simulink model "MotorTorqueControlTest_working_5_8_2022_ADC_FILT_Mo"  (R2024b)
settings: Solver=FixedStepAuto  StartTime=0.0  StopTime=inf  FixedStep=0.001  RelTol=1e-3  EnableMultiTasking=on
undefined symbols (not defined in the file): mu_X, mu_y, sigma_X, sigma_y
libraries: slrealtimeethercatlib x35, slrealtimeiplib x6, slrealtimeutilitieslib x5, simulink_extras x5, slrealtimeloglib x3, slpidlib x1, simulink x1
(part 3 of 4)

== matlab function MotorTorqueControlTest_working_5_8_2022_ADC_FILT_Mo/pack_data ==
  data: p_all input; x output; IMU_all input; angle input; phase input; p_min input; p_max input
function x = pack_data(p_all, IMU_all, angle, phase, p_min, p_max)
% Compute derived pressure features


p_heel = max(p_all([2,7]));
p_arc  = p_all(5);
p_meta = max(p_all([3,4,8]));
p_toe  = max(p_all([1,6]));
p_sum = sum(p_all);

%% Normalize pressure features
denom = p_max - p_min;
p_heel_norm = (p_heel - p_min) / denom;
p_arc_norm  = (p_arc  - p_min) / denom;
p_meta_norm = (p_meta - p_min) / denom;
p_toe_norm  = (p_toe  - p_min) / denom;
p_sum_norm = (p_sum - p_min) / denom;



% Compute acceleration magnitude (aM) from IMU measurements (assume first three are acceleration)
aM = sqrt(sum(IMU_all(1:3).^2));

% x = [angle, p_heel_norm, p_arc_norm, p_meta_norm, p_toe_norm, p_sum_norm, IMU_all(1), IMU_all(2), IMU_all(3), aM, phase]';

% x = [angle, p_heel_norm, p_arc_norm, p_meta_norm, p_toe_norm, p_sum_norm, IMU_all(2), phase]';
x = [p_heel_norm, p_arc_norm, p_meta_norm, p_toe_norm, p_sum_norm, IMU_all(2), phase]';

== matlab function MotorTorqueControlTest_working_5_8_2022_ADC_FILT_Mo/MATLAB Function ==
  data: SV_target_curr input; SV_target_next output; Uc_all_one input; Uc_non_one input; step_up input; step_down input; SV_target_min input; SV_target_max input; heel_strike input; assist_level input; min_cycles input; assist_threshold input
function SV_target_next = update_target_sv( ...
    SV_target_curr, ...
    Uc_all_one, Uc_non_one, ...
    step_up, step_down, ...
    SV_target_min, SV_target_max, ...
    heel_strike, ...
    assist_level, ...
    min_cycles, ...
    assist_threshold) %#codegen

    persistent cycles_assist

    if isempty(cycles_assist)
        cycles_assist = 0;
    end

    SV_target_next = SV_target_curr;

    if heel_strike == 0
        return
    end

    % Update internal assistance-cycle counter at heel strike
    if assist_level > assist_threshold
        cycles_assist = cycles_assist + 1;
    else
        cycles_assist = 0;
    end

    % Increase rule remains unchanged
    if Uc_all_one > 0.5
        SV_target_next = SV_target_curr + step_up;

    % Decrease only allowed if assistance has remained above
    % assist_threshold for at least min_cycles cycles
    elseif Uc_non_one > 0.5 && cycles_assist >= min_cycles
        SV_target_next = SV_target_curr - step_down;
    end

    % Clamp to bounds
    if SV_target_next > SV_target_max
        SV_target_next = SV_target_max;
    elseif SV_target_next < SV_target_min
        SV_target_next = SV_target_min;
    end
end

== matlab function MotorTorqueControlTest_working_5_8_2022_ADC_FILT_Mo/SV Estimator/circBuffer2 ==
  data: updated_SV output; SV input; heel_strike input
function updated_SV = circbuffer(SV, heel_strike)
%#codegen
% SV          : current sample value (scalar)
% heel_strike : logical/boolean flag
% updated_SV  : mean of 2-sample circular buffer

    persistent buf idx
    
    % Initialize persistent variables on first call
    if isempty(buf)
        % 2‑element buffer, same type as SV
        buf = zeros(1, 30, 'like', SV);
        idx = 1;
    end

    % Update buffer only on heel strike
    if heel_strike
        buf(idx) = SV;
        idx = rem(idx, 2) + 1;   % cycles 1 → 2 → 1 → 2 ...
    end

    % Output mean of buffer
    % (equivalent to mean(buf) but explicit for clarity)
    updated_SV = (buf(1) + buf(2)) / 2;
end

== matlab function MotorTorqueControlTest_working_5_8_2022_ADC_FILT_Mo/MATLAB Function3 ==
  data: Uc input; window_len_up input; window_len_down input; heel_strike input; Uc_buffer input; Uc_count input; Uc_all_one output; Uc_non_one output; Uc_buffer_next output; Uc_count_next output
function [Uc_all_one, Uc_non_one, Uc_buffer_next, Uc_count_next] = calculate_Uc_hist( ...
    Uc, window_len_up, window_len_down, heel_strike, Uc_buffer, Uc_count) %#codegen
% Uc_all_one: 1 if >=90% of last window_len_up samples are 1
% Uc_non_one: 1 if >=90% of last window_len_down samples are NOT 1
% IMPORTANT: heel_strike must be a 1-sample pulse (rising-edge event).
% Resets (buffer + BOTH counters) whenever either flag triggers (SV updated).

    % ---- Fixed output types/sizes ----
    Uc_all_one      = 0.0;
    Uc_non_one      = 0.0;

    Uc_buffer_next  = zeros(60,1,'like',Uc_buffer);
    Uc_buffer_next(:) = Uc_buffer(1:60);

    Uc_count_next   = zeros(2,1,'like',Uc_count);
    Uc_count_next(:)= Uc_count(1:2);

    % ---- Clamp window lengths to [1,60] ----
    Nup = int32(floor(window_len_up));
    if Nup < 1,  Nup = int32(1);  elseif Nup > 60, Nup = int32(60); end

    Ndn = int32(floor(window_len_down));
    if Ndn < 1,  Ndn = int32(1);  elseif Ndn > 60, Ndn = int32(60); end

    % ---- Use ONE shared count (stored in both elements for compatibility) ----
    count = int32(Uc_count_next(1));
    if count < 0
        count = int32(0);
    elseif count > 60
        count = int32(60);
    end

    % ---- Update buffer + count ONLY at heel strike pulse ----
    if heel_strike ~= 0
        Uc_buffer_next(1:end-1) = Uc_buffer_next(2:end);
        Uc_buffer_next(end)     = Uc;

        if count < 60
            count = count + 1;
        end
    end

    % Write count back (both entries same)
    Uc_count_next(1) = cast(count,'like',Uc_count_next(1));
    Uc_count_next(2) = cast(count,'like',Uc_count_next(2));

    tol = 1e-6; % if your Uc is "almost 1" (e.g., 0.999), increase this (e.g., 1e-3)

    % ---- Evaluate BOTH flags from the same buffer snapshot ----
    trig_up = false;
    trig_dn = false;

    % ===== UP: all-one =====
    if count >= Nup
        idx0 = int32(61) - Nup;       % 60 - Nup + 1
        oneCount = int32(0);
        for i = idx0:int32(60)
            if Uc_buffer_next(i) >= (1 - tol)
                oneCount = oneCount + 1;
            end
        end
        need90 = idivide(int32(9)*Nup + int32(9), int32(10), 'floor'); % ceil(0.9*Nup)
        if oneCount >= need90
            Uc_all_one = 1.0;
            trig_up = true;
        end
    end

    % ===== DOWN: non-one =====
    if count >= Ndn
        idx0 = int32(61) - Ndn;
        oneCount = int32(0);
        for i = idx0:int32(60)
            if Uc_buffer_next(i) >= (1 - tol)
                oneCount = oneCount + 1;
            end
        end
        need90 = idivide(int32(9)*Ndn + int32(9), int32(10), 'floor'); % ceil(0.9*Ndn)
        if (Ndn - oneCount) >= need90
            Uc_non_one = 1.0;
            trig_dn = true;
        end
    end

    % ---- Reset AFTER any trigger (SV updated), regardless of direction ----
    if trig_up || trig_dn
        Uc_buffer_next(:) = 0;
        count = int32(0);
        Uc_count_next(1) = cast(count,'like',Uc_count_next(1));
        Uc_count_next(2) = cast(count,'like',Uc_count_next(2));
    end
end

== matlab function MotorTorqueControlTest_working_5_8_2022_ADC_FILT_Mo/update_target_sv_mean_assistance ==
  data: SV_target_curr input; SV_target_next output; Uc_all_one input; Uc_non_one input; step_up input; step_down input; SV_target_min input; SV_target_max input; heel_strike input; assist_level input; min_cycles input; assist_threshold input
function SV_target_next = update_target_sv( ...
    SV_target_curr, ...
    Uc_all_one, Uc_non_one, ...
    step_up, step_down, ...
    SV_target_min, SV_target_max, ...
    heel_strike, ...
    assist_level, ...
    min_cycles, ...
    assist_threshold) %#codegen

    persistent assist_hist hist_count

    if isempty(assist_hist)
        assist_hist = zeros(30,1);   % store up to last 30 cycles
        hist_count   = 0;
    end

    SV_target_next = SV_target_curr;

    if heel_strike == 0
        return
    end

    % Make sure min_cycles stays within valid range [1, 30]
    window_len = round(min_cycles);
    if window_len < 1
        window_len = 1;
    elseif window_len > 30
        window_len = 30;
    end

    % Update assistance history at heel strike
    if hist_count < 30
        hist_count = hist_count + 1;
        assist_hist(hist_count) = assist_level;
    else
        assist_hist(1:29) = assist_hist(2:30);
        assist_hist(30)   = assist_level;
    end

    % Increase rule remains unchanged
    if Uc_all_one > 0.5
        SV_target_next = SV_target_curr + step_up;

    % Decrease rule uses mean of last min_cycles assistance values
    elseif Uc_non_one > 0.5 && hist_count >= window_len
        sum_assist = 0;
        for k = hist_count-window_len+1 : hist_count
            sum_assist = sum_assist + assist_hist(k);
        end
        mean_assist = sum_assist / window_len;

        if mean_assist > assist_threshold
            SV_target_next = SV_target_curr - step_down;
        end
    end

    % Clamp to bounds
    if SV_target_next > SV_target_max
        SV_target_next = SV_target_max;
    elseif SV_target_next < SV_target_min
        SV_target_next = SV_target_min;
    end
end

== matlab function MotorTorqueControlTest_working_5_8_2022_ADC_FILT_Mo/MATLAB Function1 ==
  data: heel_strike input; error input; gamma input; a output; gain input; a input
function a = ILC(heel_strike, error, gamma, gain, a)
    if heel_strike
        error = max(0, error);
        a = gamma * a + gain * error;
    
        if a > 10
            a = 10;
        elseif a < 0
            a = 0;
        end
    end
end

== matlab function MotorTorqueControlTest_working_5_8_2022_ADC_FILT_Mo/SV Estimator/SV_Estimator1 ==
  data: curTime input; strideSV output; data input; data_filtered input; SL output; thr_sum_FC input; thr_sum_LC input; min_event_dt input; pSum output; reset input; is_active output
function [strideSV, SL, pSum, is_active] = ...
    SV_Estimator(curTime, data, data_filtered, ...
                 thr_sum_FC, thr_sum_LC, ...
                 min_event_dt, reset) %#codegen
% Online stride-velocity estimator (pressure envelope + minAcc ZUPT)
%
% INPUT
%   data         : row-vector (width ≥ 14). May be single or double.
%                  data(1)     = time stamp (s)
%                  data(12:14) = IMU accel channels (device frame)
%   data_filtered: row-vector with pressure channels in 1:8 (here)
%   thr_sum_FC   : threshold on pSum for foot contact (FC)
%   thr_sum_LC   : threshold on pSum for foot off / load removal (LC)
%   min_event_dt : minimum time between FC / LC events (s)
%   reset        : scalar logical/0-1. When non-zero, ALL internal state is reset.
%
% OUTPUT
%   strideSV     : stride-mean velocity (m/s)
%   SL           : stride length (m)
%   pSum         : current pressure envelope (for plotting/tuning)
%   is_active    : logical flag, 1 when current estimate is considered usable.
%                  After any reset or error, this stays 0 for 3 calls.

% ------------------------------------------------------------------
% default outputs
strideSV  = 0.0;
SL        = 0.0;
pSum      = 0.0;
is_active = false;

% ------------------------------------------------------------------
% fixed parameters (internal)
g_NJ         = 9.80665;      % gravity (m/s²)
BUFFER       = 5000;         % ring-buffer length
MAX_STRIDE_T = 3.0;          % max LC→LC stride time (s)
ALPHA_FF     = 0.6;          % fraction of stance peak for FF gate
SEP_MIN      = 0.50;         % min time separation for FC/LC FSM transitions
MAX_SV       = 2.0;          % reset if strideSV > 2 m/s (safety)

% external reset flag for this call
doReset = (reset ~= 0);

% ------------------------------------------------------------------
% persistent state
persistent buf               % 11 × BUFFER: accel, vel, pos, time
persistent pEnvBuf           % 1 × BUFFER : pressure envelope (pSum)
persistent iter
persistent FC_iter LC_iter
persistent FC_idx  LC_idx
persistent SL_p strideSV_p
persistent pSum_prev tFC tLC
persistent cooldownSteps     % ≥0: remaining steps where is_active = false

% buf rows
ROW_AX=1; ROW_AY=2; ROW_AZ=3; ROW_AM=4;
ROW_VX=5; ROW_VY=6; ROW_VZ=7;
ROW_PX=8; ROW_PY=9; ROW_PZ=10; ROW_T=11;

% ------------------------------------------------------------------
% FIRST-CALL OR EXTERNAL RESET INITIALIZATION
if isempty(iter) || doReset
    buf      = zeros(11,BUFFER);
    pEnvBuf  = zeros(1,BUFFER);
    iter     = 1;

    FC_iter  = 0;
    LC_iter  = 0;
    FC_idx   = ones(1,2);
    LC_idx   = ones(1,2);

    SL_p       = 0;
    strideSV_p = 0;

    pSum_prev  = 0;
    tFC        = [-inf -inf];
    tLC        = [-inf -inf];

    % start (or restart) 3-step inactive window after reset
    cooldownSteps = 3;
end

% ------------------------------------------------------------------
% decode current packet (pressure + accel)
pressure = double(data_filtered);
IMU_data = double(data);

% keep the same heel/toe grouping for pSum as your original code
pHeel = max( pressure([2 7 8]) );
pToe  = max( pressure([1 3 4 5 6]) );
pSum  = pHeel + 1.5 * pToe;      % envelope

ax = -IMU_data(3);
ay =  IMU_data(1);
az = -IMU_data(2);

% ------------------------------------------------------------------
% gait-event detector (FC/LC from pSum)
isFC = (pSum_prev <= thr_sum_FC) && (pSum >  thr_sum_FC) ...
       && (curTime - tFC(2) > min_event_dt);
isLC = (pSum_prev >  thr_sum_LC) && (pSum <= thr_sum_LC) ...
       && (curTime - tLC(2) > min_event_dt);

if isFC
    tFC = [tFC(2) curTime];
end
if isLC
    tLC = [tLC(2) curTime];
end

pSum_prev = pSum;

% ------------------------------------------------------------------
% store current sample in buffers
idx = iter;

axg = ax * g_NJ;
ayg = ay * g_NJ;
azg = az * g_NJ;

buf(ROW_AX,idx) = axg;
buf(ROW_AY,idx) = ayg;
buf(ROW_AZ,idx) = azg;
buf(ROW_AM,idx) = sqrt(axg*axg + ayg*ayg + azg*azg);
buf(ROW_T ,idx) = curTime;

pEnvBuf(idx) = pSum;

% ------------------------------------------------------------------
% update simple FC / LC finite-state machines
if isFC
    if FC_iter==0
        FC_idx(1) = idx;
        FC_iter   = 1;
    elseif FC_iter==1 && (curTime - buf(ROW_T,FC_idx(1)) > SEP_MIN)
        FC_idx(2) = idx;
        FC_iter   = 2;
    elseif FC_iter==2 && (curTime - buf(ROW_T,FC_idx(2)) > SEP_MIN)
        FC_idx(1) = idx;
        FC_iter   = 1;
        LC_iter   = 0;
    end
end

if isLC && FC_iter>=1
    if LC_iter==0
        LC_idx(1) = idx;
        LC_iter   = 1;
    elseif LC_iter==1 && (curTime - buf(ROW_T,LC_idx(1)) > SEP_MIN)
        LC_idx(2) = idx;
        LC_iter   = 2;
    elseif LC_iter==2 && (curTime - buf(ROW_T,LC_idx(2)) > SEP_MIN)
        FC_iter   = 0;
        LC_iter   = 0;
    end
end

% ------------------------------------------------------------------
% stride finished?  (two FCs and two LCs available)
if FC_iter==2 && LC_iter==2
    fc0 = FC_idx(1); fc1 = FC_idx(2);
    lc0 = LC_idx(1); lc1 = LC_idx(2);

    % LC-to-LC stride duration
    dtLC = buf(ROW_T,lc1) - buf(ROW_T,lc0);

    % sanity check on stride duration
    if dtLC <= 0 || dtLC > MAX_STRIDE_T
        % invalid stride: don't update SL_p / strideSV_p, reset FSM
        FC_iter = 0;
        LC_iter = 0;

        % mark error → 3-step inactive window
        cooldownSteps = 3;

    else
        % ----------------------------------------------------------
        % 1) compute stance peaks for each stance (fc0→lc0, fc1→lc1)
        pPeak0 = 0;
        k      = fc0;
        while true
            v = pEnvBuf(k);
            if v > pPeak0
                pPeak0 = v;
            end
            if k == lc0, break; end
            k = adv(k, BUFFER);
        end

        pPeak1 = 0;
        k      = fc1;
        while true
            v = pEnvBuf(k);
            if v > pPeak1
                pPeak1 = v;
            end
            if k == lc1, break; end
            k = adv(k, BUFFER);
        end

        thrFF0 = ALPHA_FF * pPeak0;
        thrFF1 = ALPHA_FF * pPeak1;

        % 2) pick ZUPT indices using minAcc inside high-pressure window
        [sIdx, ~] = minAccIdxHighP(fc0, lc0, thrFF0, buf, pEnvBuf, ROW_AM, BUFFER);
        [eIdx, ~] = minAccIdxHighP(fc1, lc1, thrFF1, buf, pEnvBuf, ROW_AM, BUFFER);

        % ----------------------------------------------------------
        % ORIGINAL-STYLE 2-PASS INTEGRATION WITH DRIFT REMOVAL

        % zero velocity & position at integration start
        buf(ROW_VX,sIdx) = 0;
        buf(ROW_VY,sIdx) = 0;
        buf(ROW_VZ,sIdx) = 0;
        buf(ROW_PX,sIdx) = 0;
        buf(ROW_PY,sIdx) = 0;
        buf(ROW_PZ,sIdx) = 0;

        % first pass: accel → vel
        p = sIdx;
        c = adv(p, BUFFER);
        while true
            dt_loc = buf(ROW_T,c) - buf(ROW_T,p);
            buf(ROW_VX,c) = buf(ROW_VX,p) + 0.5*(buf(ROW_AX,p)+buf(ROW_AX,c))*dt_loc;
            buf(ROW_VY,c) = buf(ROW_VY,p) + 0.5*(buf(ROW_AY,p)+buf(ROW_AY,c))*dt_loc;
            buf(ROW_VZ,c) = buf(ROW_VZ,p) + 0.5*(buf(ROW_AZ,p)+buf(ROW_AZ,c))*dt_loc;
            if c == eIdx, break; end
            p = c;
            c = adv(c, BUFFER);
        end

        dtStride = buf(ROW_T,eIdx) - buf(ROW_T,sIdx);
        if dtStride == 0
            dtStride = eps;
        end

        vxD = buf(ROW_VX,eIdx) / dtStride;
        vyD = buf(ROW_VY,eIdx) / dtStride;
        vzD = buf(ROW_VZ,eIdx) / dtStride;

        % second pass: subtract linear drift, vel → pos
        p = sIdx;
        c = adv(p, BUFFER);
        while true
            dt_loc = buf(ROW_T,c) - buf(ROW_T,p);
            tOff   = buf(ROW_T,c) - buf(ROW_T,sIdx);

            buf(ROW_VX,c) = buf(ROW_VX,c) - vxD*tOff;
            buf(ROW_VY,c) = buf(ROW_VY,c) - vyD*tOff;
            buf(ROW_VZ,c) = buf(ROW_VZ,c) - vzD*tOff;

            buf(ROW_PX,c) = buf(ROW_PX,p) + 0.5*(buf(ROW_VX,p)+buf(ROW_VX,c))*dt_loc;
            buf(ROW_PY,c) = buf(ROW_PY,p) + 0.5*(buf(ROW_VY,p)+buf(ROW_VY,c))*dt_loc;
            buf(ROW_PZ,c) = buf(ROW_PZ,p) + 0.5*(buf(ROW_VZ,p)+buf(ROW_VZ,c))*dt_loc;

            if c == eIdx, break; end
            p = c;
            c = adv(c, BUFFER);
        end

        % stride length & mean velocity
        SL_p       = sqrt(buf(ROW_PX,eIdx)^2 + buf(ROW_PY,eIdx)^2 + buf(ROW_PZ,eIdx)^2);
        strideSV_p = SL_p / dtLC;
        if strideSV_p < 0
            strideSV_p = 0;
        end

        % optional hard reset on absurdly large SV
        if strideSV_p > MAX_SV
            buf(:,:)   = 0;
            pEnvBuf(:) = 0;
            iter       = 1;

            FC_iter  = 0;
            LC_iter  = 0;
            FC_idx   = ones(1,2);
            LC_idx   = ones(1,2);

            SL_p       = 0;
            strideSV_p = 0;

            pSum_prev  = 0;
            tFC        = [-inf -inf];
            tLC        = [-inf -inf];

            % hard error reset → 3-step inactive window
            cooldownSteps = 3;
        else
            % shift FC/LC indices for next stride
            FC_idx(1) = FC_idx(2);
            FC_iter   = 1;
            LC_idx(1) = LC_idx(2);
            LC_iter   = 1;
        end
    end
end

% advance iterator in ring buffer
iter = iter + 1;
if iter > BUFFER
    iter = 1;
end

% ------------------------------------------------------------------
% update activity flag: 3-sample cooldown after reset/error
if isempty(cooldownSteps)
    cooldownSteps = 0;
end

if cooldownSteps > 0
    is_active     = false;
    cooldownSteps = cooldownSteps - 1;
else
    is_active = true;
end

% ------------------------------------------------------------------
% outputs from persistent state
strideSV = strideSV_p;
SL       = SL_p;

end  % main function

% ==================================================================
% Helper: advance index in ring buffer
function n = adv(i, BUFFER)
n = i + 1;
if n > BUFFER
    n = 1;
end
end

% ==================================================================
% Helper: min acceleration magnitude in high-pressure window
function [idxOut, usedHigh] = minAccIdxHighP(iStart, iEnd, thrP, buf, pEnvBuf, ROW_AM, BUFFER)
% Find contiguous high-pressure window and pick min|a| inside it.
% If none exists, fall back to pure minAcc over [iStart, iEnd].

% 1) Find first and last indices with pEnv > thrP
found     = false;
firstHigh = iStart;
lastHigh  = iStart;

idx = iStart;
while true
    pEnv = pEnvBuf(idx);
    if pEnv > thrP
        if ~found
            firstHigh = idx;
            found     = true;
        end
        lastHigh = idx;
    end
    if idx == iEnd, break; end
    idx = adv(idx, BUFFER);
end

if found
    % 2) min |a| inside [firstHigh, lastHigh]
    idxOut   = firstHigh;
    mAcc     = buf(ROW_AM,idxOut);
    usedHigh = true;

    idx = firstHigh;
    while true
        accMag = buf(ROW_AM,idx);
        if accMag < mAcc
            mAcc   = accMag;
            idxOut = idx;
        end
        if idx == lastHigh, break; end
        idx = adv(idx, BUFFER);
    end
else
    % 3) fallback: no high-pressure region → minAcc over whole FC-LC
    idxOut   = minAccIdx(iStart,iEnd,buf,ROW_AM,BUFFER);
    usedHigh = false;
end
end

% ==================================================================
% Helper: pure minimum acceleration magnitude between iStart and iEnd
function idxOut = minAccIdx(iStart, iEnd, buf, ROW_AM, BUFFER)
idx    = iStart;
idxOut = iStart;
mAcc   = buf(ROW_AM,idx);

while true
    accMag = buf(ROW_AM,idx);
    if accMag < mAcc
        mAcc   = accMag;
        idxOut = idx;
    end
    if idx == iEnd, break; end
    idx = adv(idx, BUFFER);
end
end

== matlab function MotorTorqueControlTest_working_5_8_2022_ADC_FILT_Mo/Stall Check ==
  data: torque_actual input; Start_Stop input; status output; isAlive output
function [status, isAlive] = TorqueWatchdog(torque_actual, Start_Stop)
% status  : 1 = stream alive, 0 = stopped or stalled
% isStall : 1 = stall detected (latched), 0 = no stall yet
%
% Uses numeric 0/1 only (no logical true/false keywords).
% Outputs are type DOUBLE to match Simulink’s default.
%
%#codegen

% ----- USER‑TUNABLE CONSTANTS -----
Ts        = 0.001;   % sample time [s]  (set to your model step)
stallTime = 0.05;    % flat‑line duration to declare stall [s]
epsTorque = 0.000006;    % minimum change that counts as “different”
% ----------------------------------

% Persistent state
persistent lastTorque timeFrozen stallDetected sensorReady
if isempty(lastTorque)
    lastTorque     = torque_actual; % initial value
    timeFrozen     = 0;
    stallDetected  = 0;   % 0 = not stalled, 1 = stalled
    sensorReady    = 0;   % 0 = waiting for first non‑zero change
end

% ----- master gate -----
if Start_Stop == 0          % external stop / reset
    status        = 0;
    isAlive       = 1;
    timeFrozen    = 0;
    stallDetected = 0;
    sensorReady   = 0;
    lastTorque    = torque_actual;
    return
end

% ----- Start_Stop == 1 -----
if sensorReady == 0         % ignore initial flat‑line until sensor moves
    if abs(torque_actual - lastTorque) > epsTorque
        sensorReady = 1;    % sensor awake
        timeFrozen  = 0;
    end
    status  = 1;            % considered alive during warm‑up
else                         % normal watchdog
    if stallDetected == 1
        status = 0;         % latched stall
    else
        if abs(torque_actual - lastTorque) < epsTorque
            timeFrozen = timeFrozen + Ts;
            if timeFrozen >= stallTime
                stallDetected = 1;
            end
        else
            timeFrozen = 0;  % any change resets timer
        end
        status = 1 - stallDetected;  % 1 if not stalled, 0 if stalled
    end
end

% second output
isAlive = 1 - stallDetected;

% update history
lastTorque = torque_actual;
end

== matlab function MotorTorqueControlTest_working_5_8_2022_ADC_FILT_Mo/MATLAB Function4 ==
  data: x input; y output; mu_X input; sigma_X input; mu_y input; add_mu_y input; sigma_y input
function y = callGP(x, mu_X, sigma_X, mu_y, add_mu_y, sigma_y)
%#codegen
y = myModelPredict(x, mu_X, sigma_X, mu_y + add_mu_y, sigma_y);

== matlab function MotorTorqueControlTest_working_5_8_2022_ADC_FILT_Mo/SV Estimator/SV_Estimator ==
  data: curTime input; strideSV output; data input; data_filtered input; SL output; thr_sum_FC input; thr_sum_LC input; min_event_dt input; pSum output; reset input; is_active output
function [strideSV, SL, pSum, is_active] = ...
    SV_Estimator(curTime, data, data_filtered, ...
                 thr_sum_FC, thr_sum_LC, ...
                 min_event_dt, reset) %#codegen
% Online stride-velocity estimator (pressure envelope + minAcc ZUPT)
%
% INPUT
%   data         : row-vector (width ≥ 14). May be single or double.
%                  data(1)     = time stamp (s)
%                  data(12:14) = IMU accel channels (device frame)
%   data_filtered: row-vector with pressure channels in 1:8 (here)
%   thr_sum_FC   : threshold on pSum for foot contact (FC)
%   thr_sum_LC   : threshold on pSum for foot off / load removal (LC)
%   min_event_dt : minimum time between FC / LC events (s)
%   reset        : scalar logical/0-1. When non-zero, ALL internal state is reset.
%
% OUTPUT
%   strideSV     : stride-mean velocity (m/s). Updated only on a plausible
%                  stride; otherwise HOLDS the previous good value.
%   SL           : stride length (m)
%   pSum         : current pressure envelope (for plotting/tuning)
%   is_active    : logical flag, 1 when current estimate is considered usable.
%                  After any reset or error, this stays 0 for 3 calls.

% ------------------------------------------------------------------
% default outputs
strideSV  = 0.0;
SL        = 0.0;
pSum      = 0.0;
is_active = false;

% ------------------------------------------------------------------
% fixed parameters (internal)
g_NJ         = 9.80665;      % gravity (m/s²)
BUFFER       = 5000;         % ring-buffer length
MAX_STRIDE_T = 3.0;          % max LC→LC stride time (s)
ALPHA_FF     = 0.6;          % fraction of stance peak for FF gate
SEP_MIN      = 0.50;         % min time separation for FC/LC FSM transitions

% >>> CHANGED (1): plausibility band replaces the MAX_SV hard-reset.
% A stride whose estimated velocity is outside this band is treated as a bad
% estimate: the estimator HOLDS its previous good output instead of publishing
% the bad value (and instead of the old reset that zeroed the output and caused
% the drop-outs to 0). The downstream smoothing block is unchanged, so the
% controller keeps the same responsiveness -- it just never sees a bad stride.
% Set SV_MAX_VALID a little above the fastest speed the wearer actually walks.
SV_MIN_VALID = 0.3;          % m/s : below this -> integration collapsed, reject
SV_MAX_VALID = 1.8;          % m/s : above this -> integration blew up,  reject

% external reset flag for this call
doReset = (reset ~= 0);

% ------------------------------------------------------------------
% persistent state
persistent buf               % 11 × BUFFER: accel, vel, pos, time
persistent pEnvBuf           % 1 × BUFFER : pressure envelope (pSum)
persistent iter
persistent FC_iter LC_iter
persistent FC_idx  LC_idx
persistent SL_p strideSV_p
persistent pSum_prev tFC tLC
persistent cooldownSteps     % ≥0: remaining steps where is_active = false

% buf rows
ROW_AX=1; ROW_AY=2; ROW_AZ=3; ROW_AM=4;
ROW_VX=5; ROW_VY=6; ROW_VZ=7;
ROW_PX=8; ROW_PY=9; ROW_PZ=10; ROW_T=11;

% ------------------------------------------------------------------
% FIRST-CALL OR EXTERNAL RESET INITIALIZATION
if isempty(iter) || doReset
    buf      = zeros(11,BUFFER);
    pEnvBuf  = zeros(1,BUFFER);
    iter     = 1;

    FC_iter  = 0;
    LC_iter  = 0;
    FC_idx   = ones(1,2);
    LC_idx   = ones(1,2);

    SL_p       = 0;
    strideSV_p = 0;

    pSum_prev  = 0;
    tFC        = [-inf -inf];
    tLC        = [-inf -inf];

    % start (or restart) 3-step inactive window after reset
    cooldownSteps = 3;
end

% ------------------------------------------------------------------
% decode current packet (pressure + accel)
pressure = double(data_filtered);
IMU_data = double(data);

% keep the same heel/toe grouping for pSum as your original code
pHeel = max( pressure([2 7 8]) );
pToe  = max( pressure([1 3 4 5 6]) );
pSum  = pHeel + 1.5 * pToe;      % envelope

ax = -IMU_data(3);
ay =  IMU_data(1);
az = -IMU_data(2);

% ------------------------------------------------------------------
% gait-event detector (FC/LC from pSum)
isFC = (pSum_prev <= thr_sum_FC) && (pSum >  thr_sum_FC) ...
       && (curTime - tFC(2) > min_event_dt);
isLC = (pSum_prev >  thr_sum_LC) && (pSum <= thr_sum_LC) ...
       && (curTime - tLC(2) > min_event_dt);

if isFC
    tFC = [tFC(2) curTime];
end
if isLC
    tLC = [tLC(2) curTime];
end

pSum_prev = pSum;

% ------------------------------------------------------------------
% store current sample in buffers
idx = iter;

axg = ax * g_NJ;
ayg = ay * g_NJ;
azg = az * g_NJ;

buf(ROW_AX,idx) = axg;
buf(ROW_AY,idx) = ayg;
buf(ROW_AZ,idx) = azg;
buf(ROW_AM,idx) = sqrt(axg*axg + ayg*ayg + azg*azg);
buf(ROW_T ,idx) = curTime;

pEnvBuf(idx) = pSum;

% ------------------------------------------------------------------
% update simple FC / LC finite-state machines
if isFC
    if FC_iter==0
        FC_idx(1) = idx;
        FC_iter   = 1;
    elseif FC_iter==1 && (curTime - buf(ROW_T,FC_idx(1)) > SEP_MIN)
        FC_idx(2) = idx;
        FC_iter   = 2;
    elseif FC_iter==2 && (curTime - buf(ROW_T,FC_idx(2)) > SEP_MIN)
        FC_idx(1) = idx;
        FC_iter   = 1;
        LC_iter   = 0;
    end
end

if isLC && FC_iter>=1
    if LC_iter==0
        LC_idx(1) = idx;
        LC_iter   = 1;
    elseif LC_iter==1 && (curTime - buf(ROW_T,LC_idx(1)) > SEP_MIN)
        LC_idx(2) = idx;
        LC_iter   = 2;
    elseif LC_iter==2 && (curTime - buf(ROW_T,LC_idx(2)) > SEP_MIN)
        FC_iter   = 0;
        LC_iter   = 0;
    end
end

% ------------------------------------------------------------------
% stride finished?  (two FCs and two LCs available)
if FC_iter==2 && LC_iter==2
    fc0 = FC_idx(1); fc1 = FC_idx(2);
    lc0 = LC_idx(1); lc1 = LC_idx(2);

    % LC-to-LC stride duration
    dtLC = buf(ROW_T,lc1) - buf(ROW_T,lc0);

    % sanity check on stride duration
    if dtLC <= 0 || dtLC > MAX_STRIDE_T
        % invalid stride: don't update SL_p / strideSV_p, reset FSM
        FC_iter = 0;
        LC_iter = 0;

        % mark error → 3-step inactive window
        cooldownSteps = 3;

    else
        % ----------------------------------------------------------
        % 1) compute stance peaks for each stance (fc0→lc0, fc1→lc1)
        pPeak0 = 0;
        k      = fc0;
        while true
            v = pEnvBuf(k);
            if v > pPeak0
                pPeak0 = v;
            end
            if k == lc0, break; end
            k = adv(k, BUFFER);
        end

        pPeak1 = 0;
        k      = fc1;
        while true
            v = pEnvBuf(k);
            if v > pPeak1
                pPeak1 = v;
            end
            if k == lc1, break; end
            k = adv(k, BUFFER);
        end

        thrFF0 = ALPHA_FF * pPeak0;
        thrFF1 = ALPHA_FF * pPeak1;

        % 2) pick ZUPT indices using minAcc inside high-pressure window
        [sIdx, ~] = minAccIdxHighP(fc0, lc0, thrFF0, buf, pEnvBuf, ROW_AM, BUFFER);
        [eIdx, ~] = minAccIdxHighP(fc1, lc1, thrFF1, buf, pEnvBuf, ROW_AM, BUFFER);

        % ----------------------------------------------------------
        % ORIGINAL-STYLE 2-PASS INTEGRATION WITH DRIFT REMOVAL

        % zero velocity & position at integration start
        buf(ROW_VX,sIdx) = 0;
        buf(ROW_VY,sIdx) = 0;
        buf(ROW_VZ,sIdx) = 0;
        buf(ROW_PX,sIdx) = 0;
        buf(ROW_PY,sIdx) = 0;
        buf(ROW_PZ,sIdx) = 0;

        % first pass: accel → vel
        p = sIdx;
        c = adv(p, BUFFER);
        while true
            dt_loc = buf(ROW_T,c) - buf(ROW_T,p);
            buf(ROW_VX,c) = buf(ROW_VX,p) + 0.5*(buf(ROW_AX,p)+buf(ROW_AX,c))*dt_loc;
            buf(ROW_VY,c) = buf(ROW_VY,p) + 0.5*(buf(ROW_AY,p)+buf(ROW_AY,c))*dt_loc;
            buf(ROW_VZ,c) = buf(ROW_VZ,p) + 0.5*(buf(ROW_AZ,p)+buf(ROW_AZ,c))*dt_loc;
            if c == eIdx, break; end
            p = c;
            c = adv(c, BUFFER);
        end

        dtStride = buf(ROW_T,eIdx) - buf(ROW_T,sIdx);
        if dtStride == 0
            dtStride = eps;
        end

        vxD = buf(ROW_VX,eIdx) / dtStride;
        vyD = buf(ROW_VY,eIdx) / dtStride;
        vzD = buf(ROW_VZ,eIdx) / dtStride;

        % second pass: subtract linear drift, vel → pos
        p = sIdx;
        c = adv(p, BUFFER);
        while true
            dt_loc = buf(ROW_T,c) - buf(ROW_T,p);
            tOff   = buf(ROW_T,c) - buf(ROW_T,sIdx);

            buf(ROW_VX,c) = buf(ROW_VX,c) - vxD*tOff;
            buf(ROW_VY,c) = buf(ROW_VY,c) - vyD*tOff;
            buf(ROW_VZ,c) = buf(ROW_VZ,c) - vzD*tOff;

            buf(ROW_PX,c) = buf(ROW_PX,p) + 0.5*(buf(ROW_VX,p)+buf(ROW_VX,c))*dt_loc;
            buf(ROW_PY,c) = buf(ROW_PY,p) + 0.5*(buf(ROW_VY,p)+buf(ROW_VY,c))*dt_loc;
            buf(ROW_PZ,c) = buf(ROW_PZ,p) + 0.5*(buf(ROW_VZ,p)+buf(ROW_VZ,c))*dt_loc;

            if c == eIdx, break; end
            p = c;
            c = adv(c, BUFFER);
        end

        % >>> CHANGED (2): compute this stride as a CANDIDATE (local vars)
        SL_new = sqrt(buf(ROW_PX,eIdx)^2 + buf(ROW_PY,eIdx)^2 + buf(ROW_PZ,eIdx)^2);
        SV_new = SL_new / dtLC;
        if SV_new < 0
            SV_new = 0;
        end

        % >>> CHANGED (3): plausibility gate + hold-last-good
        if SV_new >= SV_MIN_VALID && SV_new <= SV_MAX_VALID
            % accept: publish this stride and roll indices to the next stride
            SL_p       = SL_new;
            strideSV_p = SV_new;

            FC_idx(1) = FC_idx(2);
            FC_iter   = 1;
            LC_idx(1) = LC_idx(2);
            LC_iter   = 1;
        else
            % reject implausible stride (collapse ~0 or blow-up):
            % HOLD the last good strideSV_p / SL_p (do NOT zero) and resync the
            % FSM, exactly like the invalid-duration path above.
            FC_iter = 0;
            LC_iter = 0;

            cooldownSteps = 3;
        end
    end
end

% advance iterator in ring buffer
iter = iter + 1;
if iter > BUFFER
    iter = 1;
end

% ------------------------------------------------------------------
% update activity flag: 3-sample cooldown after reset/error
if isempty(cooldownSteps)
    cooldownSteps = 0;
end

if cooldownSteps > 0
    is_active     = false;
    cooldownSteps = cooldownSteps - 1;
else
    is_active = true;
end

% ------------------------------------------------------------------
% outputs from persistent state
strideSV = strideSV_p;
SL       = SL_p;

end  % main function

% ==================================================================
% Helper: advance index in ring buffer
function n = adv(i, BUFFER)
n = i + 1;
if n > BUFFER
    n = 1;
end
end

% ==================================================================
% Helper: min acceleration magnitude in high-pressure window
function [idxOut, usedHigh] = minAccIdxHighP(iStart, iEnd, thrP, buf, pEnvBuf, ROW_AM, BUFFER)
% Find contiguous high-pressure window and pick min|a| inside it.
% If none exists, fall back to pure minAcc over [iStart, iEnd].

% 1) Find first and last indices with pEnv > thrP
found     = false;
firstHigh = iStart;
lastHigh  = iStart;

idx = iStart;
while true
    pEnv = pEnvBuf(idx);
    if pEnv > thrP
        if ~found
            firstHigh = idx;
            found     = true;
        end
        lastHigh = idx;
    end
    if idx == iEnd, break; end
    idx = adv(idx, BUFFER);
end

if found
    % 2) min |a| inside [firstHigh, lastHigh]
    idxOut   = firstHigh;
    mAcc     = buf(ROW_AM,idxOut);
    usedHigh = true;

    idx = firstHigh;
    while true
        accMag = buf(ROW_AM,idx);
        if accMag < mAcc
            mAcc   = accMag;
            idxOut = idx;
        end
        if idx == lastHigh, break; end
        idx = adv(idx, BUFFER);
    end
else
    % 3) fallback: no high-pressure region → minAcc over whole FC-LC
    idxOut   = minAccIdx(iStart,iEnd,buf,ROW_AM,BUFFER);
    usedHigh = false;
end
end

% ==================================================================
% Helper: pure minimum acceleration magnitude between iStart and iEnd
function idxOut = minAccIdx(iStart, iEnd, buf, ROW_AM, BUFFER)
idx    = iStart;
idxOut = iStart;
mAcc   = buf(ROW_AM,idx);

while true
    accMag = buf(ROW_AM,idx);
    if accMag < mAcc
        mAcc   = accMag;
        idxOut = idx;
    end
    if idx == iEnd, break; end
    idx = adv(idx, BUFFER);
end
end

== matlab function MotorTorqueControlTest_working_5_8_2022_ADC_FILT_Mo/MATLAB Function2 ==
  data: heel_strike input; assistance_level_new input; assistance_level input; assistance_level output
function assistance_level  = fcn(heel_strike, assistance_level_new, assistance_level)
if heel_strike
    assistance_level = assistance_level_new;
end

== matlab function MotorTorqueControlTest_working_5_8_2022_ADC_FILT_Mo/SV Estimator/Heel Strike ==
  data: is_active input; data_filtered input; heelStrike output; thr_sum input
function heelStrike = heelStrike_detect(is_active, data_filtered, thr_sum)
%#codegen
% heelStrike_detect
%   Detects heel strike based on heel pressure crossing above thr_heel.
%
% Inputs:
%   data_filtered : Nx1 vector, first 8 elements are pressures
%   thr_heel      : scalar threshold for heel pressure
%
% Output:
%   heelStrike    : logical, 1 only on the rising edge of heel contact

% --- Get heel pressure from the same channels as in calibration ---
pressure = data_filtered(1:8);
pHeel = max(pressure([2 7 8]));
pToe  = max(pressure([1 3 4 5 6]));
pSum  = pHeel + 1.5 * pToe;      % envelope

% --- Persistent state for previous heel-contact state ---
persistent prevHeelContact
if isempty(prevHeelContact)
    prevHeelContact = false;
end


% --- Define heel contact (above threshold) ---
heelContact = (pSum >= thr_sum);

if is_active
    % --- Heel strike = rising edge of heel contact ---
    heelStrike = heelContact && ~prevHeelContact;
else
    heelStrike = false;
end

% Update state
prevHeelContact = heelContact;

end

== matlab function MotorTorqueControlTest_working_5_8_2022_ADC_FILT_Mo/SV Estimator/circBuffer ==
  data: updated_SV output; SV input; heel_strike input
function updated_SV = circbuffer(SV, heel_strike)
%#codegen
% SV          : current sample value (scalar)
% heel_strike : logical/boolean flag
% updated_SV  : mean of 2-sample circular buffer

    persistent buf idx
    
    % Initialize persistent variables on first call
    if isempty(buf)
        % 2‑element buffer, same type as SV
        buf = zeros(1, 2, 'like', SV);
        idx = 1;
    end

    % Update buffer only on heel strike
    if heel_strike
        buf(idx) = SV;
        idx = rem(idx, 2) + 1;   % cycles 1 → 2 → 1 → 2 ...
    end

    % Output mean of buffer
    % (equivalent to mean(buf) but explicit for clarity)
    updated_SV = (buf(1) + buf(2)) / 2;
end

== matlab function MotorTorqueControlTest_working_5_8_2022_ADC_FILT_Mo/SV Estimator/circBuffer1 ==
  data: median_SV output; SV input; start_i input; end_i input; heel_strike input
function median_SV = circBufferMedian( ...
        SV, start_i, end_i, heel_strike) %#codegen
% SV         : current sample value
% start_i    : start index of range in circular buffer
% end_i      : end index of range in circular buffer
% heel_strike: flag indicating when to store SV
% median_SV  : median over the specified range

    N = 1000;

    % --- persistent state (no Unit Delays needed) ---------------------
    persistent buf writeIdx
    if isempty(buf)
        buf      = zeros(1, N, 'like', SV);  % circular buffer
        writeIdx = 1;                        % write index
    end

    % Fixed workspace for median calculation (local each call is fine)
    tmp = zeros(1, N, 'like', SV);

    % ------- write ----------------------------------------------------
    if heel_strike
        buf(writeIdx) = SV;
        writeIdx      = mod(writeIdx, N) + 1;
    end

    % ------- wrap indices ---------------------------------------------
    start_i = mod(start_i - 1, N) + 1;
    end_i   = mod(end_i   - 1, N) + 1;

    % ------- copy range into tmp -------------------------------------
    len = 0;
    idx = start_i;
    while true
        len        = len + 1;
        tmp(len)   = buf(idx);
        if idx == end_i
            break;
        end
        idx = idx + 1;
        if idx > N
            idx = 1;
        end
    end

    % ------- insertion sort first len elements -----------------------
    for ii = 2:len
        key = tmp(ii);
        jj  = ii - 1;
        while jj >= 1 && tmp(jj) > key
            tmp(jj + 1) = tmp(jj);
            jj = jj - 1;
        end
        tmp(jj + 1) = key;
    end

    % ------- median ---------------------------------------------------
    if mod(len, 2) ~= 0
        median_SV = tmp((len + 1) / 2);
    else
        median_SV = 0.5 * (tmp(len/2) + tmp(len/2 + 1));
    end
end

== matlab function MotorTorqueControlTest_working_5_8_2022_ADC_FILT_Mo/SV Estimator/pressure calibration ==
  data: thr_sum_out output; trigger input; data_filtered input; thr_percentage input; t input; check_window_t input
function thr_sum_out  = ...
    pressure_heel_Calib(trigger, data_filtered, thr_percentage, t, ...
                         check_window_t)
%#codegen
% trigger:        0/1
% data_filtered:  sensor data (first 8 entries are pressures)
% thr_percentage: e.g. 0.1 for 10%
% t:              current time (s)
% check_window_t: calibration window length (s)

% ---------------------------------------------------------
% 1) Compute pressures and combined channel
% ---------------------------------------------------------
pressure_all  = data_filtered(1:8);

% Example grouping of sensors into 3 channels
p1 = max(pressure_all([2 7 8]));      % channel 1
p2 = max(pressure_all([1,3,4,5,6]));  % channel 2
p3 = p1 + 1.5 * p2;                   % combined / sum channel

% 3x1 pressure vector
pressure = double(p3);

% ---------------------------------------------------------
% 2) Persistent state (replaces Unit Delays)
% ---------------------------------------------------------
persistent min_val max_val isActive startTime prevTrig
if isempty(min_val)
    % Initial values (before first calibration)
    min_val   = 0;
    max_val   = 0;
    isActive  = false;
    startTime = 0;
    prevTrig  = false;
end

% Current trigger as logical
currTrig = (trigger ~= 0);

% Rising edge: current HIGH, previous LOW
isRising = currTrig && ~prevTrig;

% ---------------------------------------------------------
% 3) Calibration window logic using persistent state
% ---------------------------------------------------------
% Handle rising edge: start (or restart) window
if isRising
    isActive  = true;
    startTime = t;
    min_val   = pressure;   % reset min to current pressures
    max_val   = pressure;   % reset max to current pressures
end

% If active, update min/max until window elapsed
if isActive
    if (t - startTime) <= check_window_t
        % Element-wise running min/max for the 3 channels
        min_val = min(min_val, pressure);
        max_val = max(max_val, pressure);
    else
        % After window, stop updating
        isActive = false;
    end
end

% ---------------------------------------------------------
% 4) Compute threshold for combined channel
% ---------------------------------------------------------
thr_vec     = min_val + thr_percentage * (max_val - min_val);
thr_sum_out = thr_vec;   % only use the 3rd channel (sum)

% Update stored trigger for next step
prevTrig = currTrig;
end

== matlab function MotorTorqueControlTest_working_5_8_2022_ADC_FILT_Mo/Subsystem1/Embedded MATLAB Function ==
  data: enable input; meas_pos input; est_pos output; phi input; delta_phase input; lambda input; c_kernel input; h input; P_in input; w_in input; delta_pos output; P_out output; w_out output
function [est_pos,delta_pos,P_out,w_out] = ...
    nonlin_filter(enable, meas_pos,phi,delta_phase,lambda,c_kernel,h,P_in,w_in)


if ~enable
    est_pos = meas_pos;
    delta_pos = meas_pos;
    P_out = P_in;
    w_out = w_in;
    return
end

% ITERATION LOOP

%%%%%%%%%%%%%%%%%%%%%%%%%%%%%%%%%%%%%%%%%%%%%%%%%%%%%%%%%%%%%%%%%%%%%%%%%%%
% psi is calculated for all the gaussina-like functions (all i)
psi = exp(h*(cos(repmat(phi,length(c_kernel),1)-c_kernel)-1));


%%%%%%%%%%%%%%%%%%%%%%%%%%%%%%%%%%%%%%%%%%%%%%%%%%%%%%%%%%%%%%%%%%%%%%%%%%%
% P_out = inverse covariance matrix for t+1
P_out = 1/lambda*(P_in-P_in.^2./(lambda./psi+P_in));


%%%%%%%%%%%%%%%%%%%%%%%%%%%%%%%%%%%%%%%%%%%%%%%%%%%%%%%%%%%%%%%%%%%%%%%%%%%
% w = weigths (all i) of the kernel functions

w_out = w_in + psi.*P_out.*(meas_pos-w_in);


%%%%%%%%%%%%%%%%%%%%%%%%%%%%%%%%%%%%%%%%%%%%%%%%%%%%%%%%%%%%%%%%%%%%%%%%%%%
% estimated position
est_pos = sum(psi.*w_out,1)./sum(psi,1);


%%%%%%%%%%%%%%%%%%%%%%%%%%%%%%%%%%%%%%%%%%%%%%%%%%%%%%%%%%%%%%%%%%%%%%%%%%%
% phase lead/lag

% calculate psi value for the phase lead/lag
psi_shift = exp(h*(cos(repmat(phi,length(c_kernel),1)+delta_phase-c_kernel)-1));

% calculate the estimated lead/lag position
delta_pos = sum(psi_shift.*w_out,1)./sum(psi_shift,1);

== matlab function MotorTorqueControlTest_working_5_8_2022_ADC_FILT_Mo/Subsystem1/Embedded MATLAB Function1 ==
  data: meas_pos input; parameters input; POstate_out output; POstate_in input
function POstate_out  = adaptive_osc(meas_pos,parameters,POstate_in)
% This function implements a discretized version of the simple adaptive oscillator
% for periodic profiles

% inputs: - meas_pos is the measured position
%         - POstate_in is the current state of the main adaptive oscillator
%         - parameters is the parameters vector
%         - coupling is the coupling parameter
%               0 no coupling - 1 hip coupling - 2 knee coupling - 3 hip and knee coupling -
%               4 left and right coupling - 5 all to all coupling
% outputs: - POstate_out is the updated state of the main adaptive oscillator

%% PARAMETERS
eps = parameters(1);    % coupling constant (speed of phase synchronization to F(t))
nu = parameters(2);     % integrator gain
stime = parameters(3);  % sampling time [s]
nbr_osc = 6;           % number of oscillators

%%%%%%%%%%%%%%%%%%%%%%%%%%%%%%%%%%%%%%%%%%%%%%%%%%%%%%%%%%%%%%%%%%%%%%%%%%%
%  ??? perchè ci sono 6 oscillatori ? corrispondono alle condizioni di
%  couplings? che senso ha?
%%%%%%%%%%%%%%%%%%%%%%%%%%%%%%%%%%%%%%%%%%%%%%%%%%%%%%%%%%%%%%%%%%%%%%%%%%%

%% PHASE OSCILLATOR STATE
offset  = POstate_in(1,:);              % alpha0(t)
omega   = POstate_in(2,:);              % frequency of the oscillator
if omega > 3*pi
    omega = 3/2*pi;
end

if omega < 1*pi
    omega = 3/2*pi;
end
phi     = POstate_in(3:2+nbr_osc,:);    % phase of the oscillator 
ampl    = POstate_in(3+nbr_osc:end,:);  % amplitude of the oscillator (alpha1(t))

%% ITERATION LOOP

%%%%%%%%%%%%%%%%%%%%%%%%%%%%%%%%%%%%%%%%%%%%%%%%%%%%%%%%%%%%%%%%%%%%%%%%%%%
% DEFINIGN TECHING SIGNAL
%%%%%%%%%%%%%%%%%%%%%%%%%%%%%%%%%%%%%%%%%%%%%%%%%%%%%%%%%%%%%%%%%%%%%%%%%%%
% teaching signals: F(t) = theta_measured - theta_estimated
% theta_measured = meas_pos
% theta estimated = offset + ampl * sin(phi(t))
teach_signal = meas_pos - offset - sum(ampl.*sin(phi),1);   


%%%%%%%%%%%%%%%%%%%%%%%%%%%%%%%%%%%%%%%%%%%%%%%%%%%%%%%%%%%%%%%%%%%%%%%%%%%
%  UPDATE OSCILLATOR PARAMETERS
%%%%%%%%%%%%%%%%%%%%%%%%%%%%%%%%%%%%%%%%%%%%%%%%%%%%%%%%%%%%%%%%%%%%%%%%%%%
% update phi to the current iteration:
% phi(t+1) = phi(t) + stima * (omega(t) + eps * teach_signal(t) * cos(phi(t)))
new_phi = mod( phi + stime*(repmat((1:nbr_osc)',1,1).*repmat(omega,nbr_osc,1) + eps*repmat(teach_signal,nbr_osc,1).*cos(phi)) , 2*pi);
% nota: il modo viene preso perchè phi è una fase percui deve essere
% compresa quindi per definizione tra 0 e 2*pi 

% update omega to the current iteration:
% omega(t+1) = omega(t) * stime * ( eps * teach_signal(t) * cos(phi(t)) )
new_omega = omega + stime*(eps*teach_signal.*cos(phi(1,:)));

% update the amplitide to the current iteration:
% ampl(t+1) = ampl(t) + stime * (nu * theach_signal(t) * sin (phi(t)) )
new_ampl = ampl + stime*(nu*repmat(teach_signal,nbr_osc,1).*sin(phi));

% update the offset to the current iteration:
% offset(t+1) = offset(t) + stime * ( nu * teachsignal(t) )
new_offset = offset + stime*(nu*teach_signal);

%%%%%%%%%%%%%%%%%%%%%%%%%%%%%%%%%%%%%%%%%%%%%%%%%%%%%%%%%%%%%%%%%%%%%%%%%%%
% COUPLING BETWEEN DIFFERENT JOINTS
%%%%%%%%%%%%%%%%%%%%%%%%%%%%%%%%%%%%%%%%%%%%%%%%%%%%%%%%%%%%%%%%%%%%%%%%%%%

% ATTENZIONE: qua non mi torna che si faccia la media anche su ampiezza ed
% offset dell'oscillatore infatti secondo me si introduce un errore nella
% stima (per il fatto che anca e ginocchio possono avere ampiezze diverse)
% che riduce la capacità dell'AFO di trackare il segnale


% % riga modificata da TL l' 8/8/2011
% Omega RESET:
% evita che l'scillatore sia attratto dalla frequenza 0
% se scende sotto 0.1 Hz viene riprotato a 0.8 Hz in modo secco
for i = 1:size(new_omega,1)
    for j = 1:size(new_omega,2)
        if new_omega(i,j)< (0.1*2*pi)
            new_omega(i,j) = 0.8*2*pi;
        end
    end
end
% NOTA: per come era scritta prima prevedeva di utilizzare vettori dalla
% lunghezza variabile
%
% % riga senza find 
% new_omega(new_omega<0.1*2*pi) = 0.8*2*pi;


% riga originale: 
% new_omega(find(new_omega<0.1*2*pi)) = 0.8*2*pi;

POstate_out = [new_offset; new_omega; new_phi; new_ampl];
